simulink model "step_1"  (R2020a)
settings: Solver=VariableStepAuto  StartTime=0.0  StopTime=10.01  RelTol=1e-3
settings Model: Creator=HP  LastModifiedBy=HP

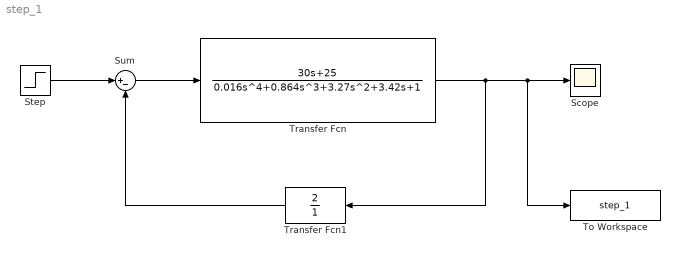
== system step_1 ==
  Scope : Scope
  Step : Step  Time=0  After=20  SampleTime=0
  Sum : Sum  Inputs=|+-
  To Workspace : ToWorkspace  VariableName=step_1  SampleTime=0.01
      settings: Save2DSignal=2-D array (concatenate along first dimension)
  Transfer Fcn : TransferFcn  Numerator=[0 0 0 30 25]  Denominator=[0.016 0.864 3.27 3.42 1]
  Transfer Fcn1 : TransferFcn  Numerator=[2]  Denominator=[1]
  wires:
  Transfer Fcn/1 -> Transfer Fcn1/1, To Workspace/1, Scope/1
  Step/1 -> Sum/1
  Sum/1 -> Transfer Fcn/1
  Transfer Fcn1/1 -> Sum/2
